simulink model "Ex5"  (R2020a)
settings: Solver=VariableStepAuto  StartTime=0.0  StopTime=10.0  RelTol=1e-3
settings Model: Creator=Joao Loureiro  LastModifiedBy=Joao Loureiro

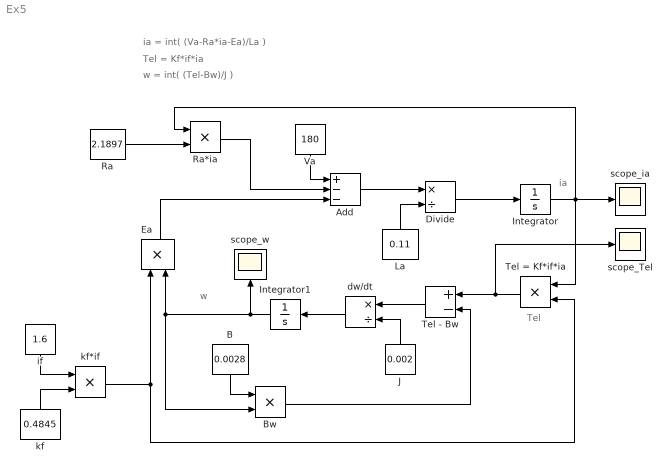
== system Ex5 ==
  note: w = int( (Tel-Bw)/J )
  note: Tel = Kf*if*ia
  note: ia = int( (Va-Ra*ia-Ea)/La )
  note: Tel
  note: w
  note: ia
  Add : Sum  Inputs=+--
  B : Constant  Value=0.0028
  Bw : Product
  Divide : Product  Inputs=*/
  Ea : Product
  Integrator : Integrator
  Integrator1 : Integrator
  J : Constant  Value=0.002
  La : Constant  Value=0.11
  Ra : Constant  Value=2.1897
  Ra*ia : Product
  Tel - Bw : Sum  Inputs=+-
  Tel = Kf*if*ia : Product
  Va : Constant  Value=180
  dw/dt : Product  Inputs=*/
  if : Constant  Value=1.6
  kf : Constant  Value=0.4845
  kf*if : Product
  scope_Tel : Scope
  scope_ia : Scope
  scope_w : Scope
  wires:
  Ra/1 -> Ra*ia/2
  Ra*ia/1 -> Add/2
  Va/1 -> Add/1
  Ea/1 -> Add/3
  Add/1 -> Divide/1
  Divide/1 -> Integrator/1
  La/1 -> Divide/2
  if/1 -> kf*if/1
  Integrator/1 -> scope_ia/1, Tel = Kf*if*ia/1, Ra*ia/1
  kf/1 -> kf*if/2
  kf*if/1 -> Ea/1, Tel = Kf*if*ia/2
  Tel = Kf*if*ia/1 -> Tel - Bw/1, scope_Tel/1
  Integrator1/1 -> Bw/2, Ea/2, scope_w/1
  J/1 -> dw/dt/2
  Tel - Bw/1 -> dw/dt/1
  dw/dt/1 -> Integrator1/1
  B/1 -> Bw/1
  Bw/1 -> Tel - Bw/2
